simulink model "observer"  (R2016b)
settings: Solver=ode45  StartTime=0.0  StopTime=10.0  RelTol=1e-3  EnableMultiTasking=on
values from neighbouring files (symbols this model uses):
  A2 = A-B*K-L*C    [LabCEE.m]
  B2 = L    [LabCEE.m]
  C2 = -K    [LabCEE.m]
  D2 = D'    [LabCEE.m]    (also in test.m)
  D3 = [D D]    [LabCEE.m]
  x_0 = [0.1 0 0 0 0]'    [LabCEE.m]    (also in test.m)
undefined symbols (not defined in the file or in its folder): A, B, C, D
settings Model: Creator=Alunos  LastModifiedBy=AndreCNF
settings DataIOCC: LimitDataPoints=on  SaveFormat=Array
settings OptimizationCC: LifeSpan=inf
settings DebuggingCC: SFUnexpectedBacktrackingDiag=warning  SFNoUnconditionalDefaultTransitionDiag=warning  SFExecutionAtInitializationDiag=none
settings HardwareCC: ProdBitPerPointer=32  ProdBitPerSizeT=32  ProdBitPerPtrDiffT=32  ProdLargestAtomicFloat=None  ProdIntDivRoundTo=Undefined  ProdEndianess=Unspecified  ProdWordSize=32  ProdHWDeviceType=32-bit Generic
settings ModelReferenceCC: PropagateSignalLabelsOutOfModel=off
settings GRTTargetCC: TargetLangStandard=C89/C90 (ANSI)  GeneratePreprocessorConditionals=Disable all
settings ConfigComp: CovMetricSettings=dw  CovHtmlReporting=on  CovSaveCumulativeToWorkspaceVar=on  CovSaveSingleToWorkspaceVar=on  CovExternalEMLEnable=off

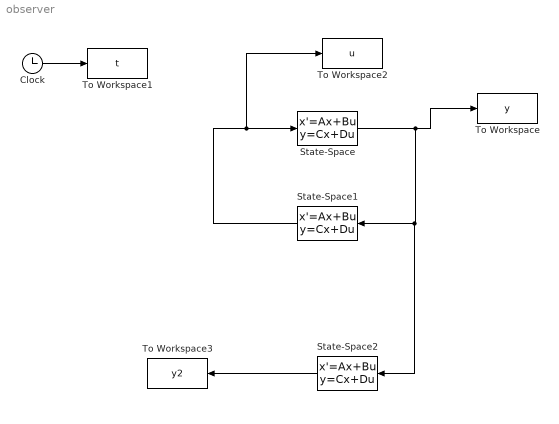
== system observer ==
  Clock : Clock
  State-Space : StateSpace  A=A  B=B  C=C  D=D  X0=x_0
  State-Space1 : StateSpace  A=A2  B=B2  C=C2  D=D2  X0=[0 0 0 0 0]
  State-Space2 : StateSpace  A=A2  B=B2  C=C  D=D3  X0=[0 0 0 0 0]
  To Workspace : ToWorkspace  VariableName=y  SampleTime=-1
  To Workspace1 : ToWorkspace  VariableName=t  SampleTime=-1
  To Workspace2 : ToWorkspace  VariableName=u  SampleTime=-1
  To Workspace3 : ToWorkspace  VariableName=y2  SampleTime=-1
  wires:
  Clock/1 -> To Workspace1/1
  State-Space/1 -> State-Space2/1, State-Space1/1, To Workspace/1
  State-Space1/1 -> To Workspace2/1, State-Space/1
  State-Space2/1 -> To Workspace3/1
